simulink model "road_profile"  (R2019a)
settings: Solver=VariableStepAuto  StartTime=0.0  StopTime=10.0  RelTol=1e-3
settings Model: Creator=Owen Heaney  LastModifiedBy=Owen Heaney

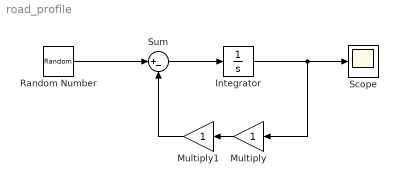
== system road_profile ==
  Integrator : Integrator
  Multiply : Gain
  Multiply1 : Gain
  Random Number : RandomNumber  SampleTime=0.1
  Scope : Scope
  Sum : Sum  Inputs=|+-
  wires:
  Random Number/1 -> Sum/1
  Sum/1 -> Integrator/1
  Integrator/1 -> Multiply/1, Scope/1
  Multiply/1 -> Multiply1/1
  Multiply1/1 -> Sum/2
